simulink model "mainModel"  (R2024b)
settings: Solver=ode4  StartTime=0.0  StopTime=35000  FixedStep=0.1  RelTol=1e-3
values from neighbouring files (symbols this model uses):
  actuators = actuatorsConfig()    [main.m]
  constant = constantsConfig()    [main.m]
  control = controlConfig(data)    [main.m]
  MEKF = estimationConfig(sensors,simOpt)    [main.m]
  pert = pertConfig()    [main.m]
  sensors = sensorsConfig()    [main.m]
undefined symbols (not defined in the file or in its folder): Ab0, data, DiscIntNeverNeededParam, init
libraries: matrix_library x38, simulink x10, aerolibutil x7, simulink_extras x6, sharedtransform x1, dspinverses x1, dspfdesign x1, dspstat3 x1
(part 3 of 3)

== system mainModel/atmDrag/trash/Relative velocity body ==
  velRel_B : Inport
  om_B : Inport  Port=2
  rF_i : Inport  Port=3
  Add : Sum  Inputs=-+
  Cross Product : matrix_library/Cross Product
  Reshape : Reshape  OutputDimensionality=Row vector (2-D)
  Reshape1 : Reshape  OutputDimensionality=Row vector (2-D)
  vRelBody : Outport
  wires:
  velRel_B/1 -> Reshape/1
  Cross Product/1 -> Add/1
  om_B/1 -> Reshape1/1
  Reshape1/1 -> Cross Product/1
  rF_i/1 -> Cross Product/2
  Add/1 -> vRelBody/1
  Reshape/1 -> Add/2

== system mainModel/atmDrag/trash/Subsystem ==
  rho : Inport
  vRelBody : Inport  Port=2
  Nb_i : Inport  Port=3
  i : Inport  Port=4
  A_i : Inport  Port=5
  Assignment1 : Assignment  Commented=on  NumberOfDimensions=2  DiagnosticForDimensions=Warning  IndexOptions=Index vector (port),Assign all  Indices=1,1  OutputSizes=1,1
  Constant5 : Constant  Commented=on  Value=zeros(length(pert.drag.A), 1)  VectorParams1D=off
  Display2 : Display  Commented=on
  Dot Product : DotProduct  OutDataTypeStr=Inherit: Inherit via internal rule
  Gain : Gain  Gain=-1/2
  Gain1 : Gain  Gain=pert.drag.CD
  Gain2 : Gain  Gain=1e3
  Product : Product  Inputs=5
  Square : Math  Operator=square
  Subsystem Reference : Subsystem  ReferencedSubsystem=vecNorm
  F_i : Outport
  dotProd : Outport  Port=2
  wires:
  Product/1 -> F_i/1, Assignment1/2  "F_i"
  Subsystem Reference/1 -> Gain2/1
  rho/1 -> Gain/1
  Gain1/1 -> Product/1
  Dot Product/1 -> Product/4, dotProd/1
  Square/1 -> Product/2
  Gain/1 -> Gain1/1
  A_i/1 -> Product/5
  Nb_i/1 -> Dot Product/2
  vRelBody/1 -> Subsystem Reference/1
  Gain2/1 -> Square/1
  Constant5/1 -> Assignment1/1
  Assignment1/1 -> Display2/1
  i/1 -> Assignment1/3
  Subsystem Reference/2 -> Dot Product/1, Product/3

== system mainModel/attitudeDetermination_QUATERNION/QUEST V2/adjointMatrix ==
  A : Inport
  Reshape : Reshape  OutputDimensionality=Customize  OutputDimensions=[3,3]
  Subsystem Reference : Subsystem  ReferencedSubsystem=matrixCoFactors
  Out1 : Outport
  wires:
  Subsystem Reference/1 -> Reshape/1
  Reshape/1 -> Out1/1
  A/1 -> Subsystem Reference/1

== system mainModel/attitudeDetermination_QUATERNION/compute Kmatrix/Kmatrix ==
  S : Inport
  z : Inport  Port=2
  sigma : Inport  Port=3
  Constant : Constant  Value=eye(3)
  Minus : Sum  Inputs=+-
  Product : Product
  To Workspace4 : ToWorkspace  VariableName=K  SampleTime=-1
  Transpose : Math  Operator=transpose
  Vector Concatenate : Concatenate  Mode=Multidimensional array  ConcatenateDimension=2
  Vector Concatenate1 : Concatenate
  Vector Concatenate2 : Concatenate  Mode=Multidimensional array
  K : Outport
  wires:
  Constant/1 -> Product/2
  sigma/1 -> Vector Concatenate1/2, Product/1
  Product/1 -> Minus/2  "sigma*I"
  S/1 -> Minus/1  "Smatrix"
  Minus/1 -> Vector Concatenate/1  "S-sigma*I"
  z/1 -> Transpose/1, Vector Concatenate/2  "zVect"
  Transpose/1 -> Vector Concatenate1/1  "zVect^t"
  Vector Concatenate1/1 -> Vector Concatenate2/2  "[zVect^t  sigma]"
  Vector Concatenate/1 -> Vector Concatenate2/1  "[S-sigmaI  zVect]"
  Vector Concatenate2/1 -> To Workspace4/1, K/1  "Kmatrix"

== system mainModel/attitudeDetermination_QUATERNION/quest - shuster/compute optimal quaternion ==
  lambda : Inport
  sigma : Inport  Port=2
  k : Inport  Port=3
  Delta : Inport  Port=4
  S : Inport  Port=5
  z : Inport  Port=6
  Subsystem : Subsystem
  Subsystem Reference : Subsystem  ReferencedSubsystem=vecNorm
  Subsystem1 : Subsystem
  Subsystem2 : Subsystem
  Subsystem3 : Subsystem
  Terminator : Terminator
  Vector Concatenate : Concatenate
  q_est : Outport
  wires:
  Subsystem2/1(X) -> Vector Concatenate/1  "qv"
  Subsystem3/1(gamma) -> Vector Concatenate/2  "qw"
  lambda/1 -> Subsystem/1(lambda), Subsystem3/2(lambda), Subsystem1/1(lambda)
  sigma/1 -> Subsystem3/3(sigma), Subsystem/2(sigma), Subsystem1/2(sigma)
  k/1 -> Subsystem/3(k)
  S/1 -> Subsystem2/2(S)
  Subsystem/1(alpha) -> Subsystem3/1(alpha), Subsystem2/3(alpha)
  Subsystem1/1(beta) -> Subsystem2/4(beta)
  z/1 -> Subsystem2/1(z)
  Delta/1 -> Subsystem3/4(Delta)
  Vector Concatenate/1 -> Subsystem Reference/1
  Subsystem Reference/2 -> q_est/1
  Subsystem Reference/1 -> Terminator/1

== system mainModel/attitudeDetermination_QUATERNION/quest - shuster/mewton method step-two ==
  lambda1 : Inport
  sigma : Inport  Port=2
  a : Inport  Port=3
  b : Inport  Port=4
  c : Inport  Port=5
  d : Inport  Port=6
  Abs : Abs  Commented=on  SaturateOnIntegerOverflow=off
  Compare To Constant : simulink/Logic and Bit Operations/Compare To Constant  Commented=on  relop=>=  const=5  OutDataTypeStr=boolean
  Scope : Scope  Commented=on
  Scope1 : Scope  Commented=on
  Switch : Switch  Commented=on  Criteria=u2 > Threshold  SaturateOnIntegerOverflow=off  InputSameDT=off
  characteristic polynomial derivative1 : Subsystem
  characteristic polynomial1 : Subsystem
  "newton method " : Subsystem
  lambda : Outport
  wires:
  lambda1/1 -> characteristic polynomial derivative1/1(lambda), characteristic polynomial1/1(lambda1), Switch/3, "newton method "/1(lambda1)
  b/1 -> characteristic polynomial derivative1/3(b), characteristic polynomial1/4(b)
  "newton method "/1(lambda) -> lambda/1, Switch/1  "lambda"
  characteristic polynomial derivative1/1(p'(lambda)) -> Abs/1, "newton method "/3(p'(lambda))
  characteristic polynomial1/1(p(lambda)) -> "newton method "/2(p(lambda))
  c/1 -> characteristic polynomial derivative1/4(c), characteristic polynomial1/5(c)
  d/1 -> characteristic polynomial1/6(d)
  sigma/1 -> characteristic polynomial1/2(sigma)
  a/1 -> characteristic polynomial derivative1/2(a), characteristic polynomial1/3(a)
  Compare To Constant/1 -> Scope1/1, Switch/2
  Switch/1 -> ?
  Abs/1 -> Scope/1, Compare To Constant/1

== system mainModel/attitudeDetermination_QUATERNION/quest - shuster/newton method step-one ==
  lambda : Inport
  sigma : Inport  Port=2
  a : Inport  Port=3
  b : Inport  Port=4
  c : Inport  Port=5
  d : Inport  Port=6
  characteristic polynomial : Subsystem
  characteristic polynomial derivative : Subsystem
  newton method step-one : Subsystem
  lambda1 : Outport
  wires:
  a/1 -> characteristic polynomial derivative/2(a), characteristic polynomial/3(a)
  newton method step-one/1(lambda1) -> lambda1/1  "lambda1"
  c/1 -> characteristic polynomial/5(c), characteristic polynomial derivative/4(c)
  sigma/1 -> characteristic polynomial/2(sigma)
  characteristic polynomial derivative/1(p'(lambda)) -> newton method step-one/2(p'(lambda))
  d/1 -> characteristic polynomial/6(d)
  characteristic polynomial/1(p(lambda)) -> newton method step-one/1(p(lambda))
  lambda/1 -> characteristic polynomial/1(lambda), characteristic polynomial derivative/1(lambda)
  b/1 -> characteristic polynomial derivative/3(b), characteristic polynomial/4(b)

== system mainModel/attitudeDetermination_QUATERNION/quest - shuster/shuster parameters ==
  S : Inport
  z : Inport  Port=2
  Sigma : Subsystem
  compute Delta : Subsystem
  compute a : Subsystem
  compute b : Subsystem
  compute c : Subsystem
  compute d : Subsystem
  compute k : Subsystem
  a : Outport
  b : Outport  Port=2
  c : Outport  Port=3
  d : Outport  Port=4
  sigma : Outport  Port=5
  k : Outport  Port=6
  Delta : Outport  Port=7
  wires:
  compute k/1(k) -> compute a/2(k), k/1
  S/1 -> compute d/1(S), compute c/3(S), compute Delta/1(S), compute k/1(S), Sigma/1(S)
  compute c/1(c) -> c/1  "c"
  z/1 -> compute d/2(z), compute c/2(z), compute b/2(z)
  compute Delta/1(Delta) -> Delta/1, compute c/1(Delta)
  compute a/1(a) -> a/1  "a"
  Sigma/1(sigma) -> compute b/1(sigma), sigma/1, compute a/1(sigma)  "sigma"
  compute b/1(b) -> b/1  "b"
  compute d/1(d) -> d/1  "d"

== system mainModel/starSensorModel/star mapping/keep3 ==
  In1 : Inport
  Abs : Abs  SaturateOnIntegerOverflow=off
  Memory : Memory  InheritSampleTime=on
  Sum of Elements1 : Sum  Inputs=+
  Switch : Switch  Criteria=u2 > Threshold  SaturateOnIntegerOverflow=off  InputSameDT=off
  s_N4 : Outport
  wires:
  Switch/1 -> s_N4/1, Memory/1
  Abs/1 -> Switch/2
  Memory/1 -> Switch/1, Sum of Elements1/1
  Sum of Elements1/1 -> Abs/1
  In1/1 -> Switch/3

== system mainModel/MEKF ESTIMATION/MEASUREMENT/KALMAN GAIN/avoid sing ==
  S : Inport
  Add : Sum
  Constant : Constant  Value=eye(6)*1e-12
  S_ : Outport
  wires:
  S/1 -> Add/2
  Constant/1 -> Add/1
  Add/1 -> S_/1

== system mainModel/MEKF ESTIMATION/MEASUREMENT/SENSITIVITY MATRIX/skewMatrix ==
  note: b_pred_skew = [0 , -b_pred(3) , b_pred(2) ;
      | b_pred(3) , 0 , -b_pred(1) ;
      | -b_pred(2) , b_pred(1) , 0 ];
  vect : Inport
  Constant : Constant  Value=0
  Demux : Demux  Outputs=3
  Gain : Gain  Gain=-1
  Gain1 : Gain  Gain=-1
  Gain2 : Gain  Gain=-1
  Reshape : Reshape  OutputDimensionality=Row vector (2-D)
  Reshape1 : Reshape  OutputDimensionality=Row vector (2-D)
  Reshape2 : Reshape  OutputDimensionality=Row vector (2-D)
  Vector Concatenate : Concatenate  NumInputs=3
  Vector Concatenate1 : Concatenate  NumInputs=3
  Vector Concatenate2 : Concatenate  NumInputs=3
  Vector Concatenate3 : Concatenate  NumInputs=3  Mode=Multidimensional array
  skew : Outport
  wires:
  Demux/1 -> Vector Concatenate2/2, Gain1/1  "x"
  Gain2/1 -> Vector Concatenate2/1
  Vector Concatenate1/1 -> Reshape1/1
  Constant/1 -> Vector Concatenate/1, Vector Concatenate1/2, Vector Concatenate2/3
  Vector Concatenate3/1 -> skew/1
  Gain/1 -> Vector Concatenate/2
  Demux/2 -> Gain2/1, Vector Concatenate/3  "y"
  Gain1/1 -> Vector Concatenate1/3
  Vector Concatenate2/1 -> Reshape2/1
  Reshape2/1 -> Vector Concatenate3/3
  Demux/3 -> Gain/1, Vector Concatenate1/1  "z"
  vect/1 -> Demux/1
  Reshape/1 -> Vector Concatenate3/1
  Vector Concatenate/1 -> Reshape/1
  Reshape1/1 -> Vector Concatenate3/2

== system mainModel/MEKF ESTIMATION/PREDICTION/STATE PROPAGATION/QUATERNION KINEMATICS ==
  q_corr : Inport
  w_corr : Inport  Port=2
  Add2 : Sum
  Constant : Constant  Value=0
  Gain : Gain  Gain=1/2
  Gain1 : Gain  Commented=on  Gain=0.5
  Gain2 : Gain  Gain=MEKF.dt
  Reshape : Reshape  OutputDimensionality=Row vector (2-D)
  Subsystem Reference : Subsystem  ReferencedSubsystem=vecNorm
  Terminator : Terminator
  Vector Concatenate : Concatenate
  q_corr x w_corr_quat : aerolibutil/Quaternion Multiplication
  quatMolt : Subsystem  Commented=on
  q_pred : Outport
  wires:
  Constant/1 -> Vector Concatenate/1
  w_corr/1 -> Vector Concatenate/2
  Vector Concatenate/1 -> quatMolt/2(In2), q_corr x w_corr_quat/2  "w_corr_quat"
  Gain2/1 -> Add2/2
  Add2/1 -> Subsystem Reference/1  "q_pred"
  q_corr/1 -> Reshape/1  "q_corr"
  Gain/1 -> Gain2/1  "qDot_pred"
  q_corr x w_corr_quat/1 -> Gain/1
  Subsystem Reference/2 -> q_pred/1
  Subsystem Reference/1 -> Terminator/1
  Reshape/1 -> Add2/1, quatMolt/1(In1), q_corr x w_corr_quat/1
  quatMolt/1(quaternions) -> Gain1/1

== system mainModel/MEKF ESTIMATION/PREDICTION/STATE PROPAGATION/SYSTEM DYNAMICS ==
  w_corr : Inport
  J : Inport  Port=2
  hWheel : Inport  Port=3
  hDotWheel : Inport  Port=4
  distTq : Inport  Port=5
  controlTq : Inport  Port=6
  Add : Sum
  Add1 : Sum  Inputs=++++
  Add2 : Sum
  Cross Product : matrix_library/Cross Product
  Cross Product1 : matrix_library/Cross Product
  Gain : Gain  Gain=-1
  Gain1 : Gain  Gain=-1
  Gain2 : Gain  Gain=MEKF.dt
  Gain3 : Gain  Gain=inv(data.Imatrix)  Multiplication=Matrix(K*u)
  Product : Product  Multiplication=Matrix(*)
  Reshape : Reshape  OutputDimensionality=Column vector (2-D)
  Reshape4 : Reshape
  w_pred : Outport
  wires:
  Product/1 -> Cross Product/2  "J*w"
  Add1/1 -> Gain3/1  "totalTq"
  Gain2/1 -> Add2/2
  J/1 -> Product/1  "J"
  w_corr/1 -> Reshape/1  "w_corr"
  Gain3/1 -> Gain2/1  "wDot_pred"
  Cross Product1/1 -> Add/2  "w x h"
  Add/1 -> Gain/1  "gyro"
  Gain/1 -> Reshape4/1
  Cross Product/1 -> Add/1  "w x Jw"
  Add2/1 -> w_pred/1  "w_pred"
  hDotWheel/1 -> Gain1/1  "hDot"
  hWheel/1 -> Cross Product1/2  "h"
  Reshape/1 -> Add2/1, Cross Product/1, Product/2, Cross Product1/1
  controlTq/1 -> Add1/4
  distTq/1 -> Add1/3
  Gain1/1 -> Add1/2
  Reshape4/1 -> Add1/1

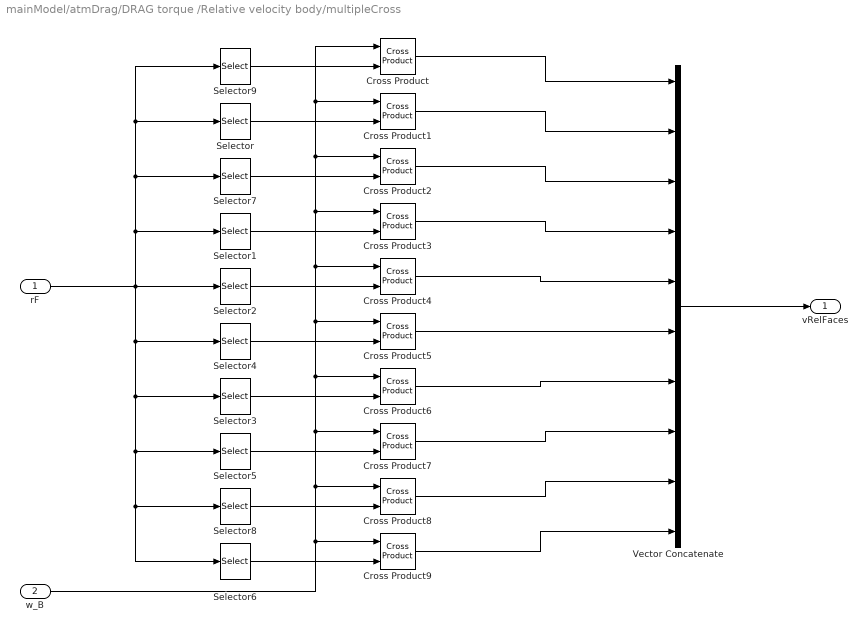
== system mainModel/atmDrag/DRAG torque /Relative velocity body/multipleCross ==
  rF : Inport
  w_B : Inport  Port=2
  Cross Product{,1..9} (10 alike) : matrix_library/Cross Product
  Selector : Selector  NumberOfDimensions=2  InputPortWidth=3  IndexOptions=Index vector (dialog),Select all  Indices=2,[1:3]  OutputSizes=1,1
  Selector1 : Selector  NumberOfDimensions=2  InputPortWidth=3  IndexOptions=Index vector (dialog),Select all  Indices=4,[1:3]  OutputSizes=1,1
  Selector2 : Selector  NumberOfDimensions=2  InputPortWidth=3  IndexOptions=Index vector (dialog),Select all  Indices=5,[1:3]  OutputSizes=1,1
  Selector3 : Selector  NumberOfDimensions=2  InputPortWidth=3  IndexOptions=Index vector (dialog),Select all  Indices=7,[1:3]  OutputSizes=1,1
  Selector4 : Selector  NumberOfDimensions=2  InputPortWidth=3  IndexOptions=Index vector (dialog),Select all  Indices=6,[1:3]  OutputSizes=1,1
  Selector5 : Selector  NumberOfDimensions=2  InputPortWidth=3  IndexOptions=Index vector (dialog),Select all  Indices=8,[1:3]  OutputSizes=1,1
  Selector6 : Selector  NumberOfDimensions=2  InputPortWidth=3  IndexOptions=Index vector (dialog),Select all  Indices=10,[1:3]  OutputSizes=1,1
  Selector7 : Selector  NumberOfDimensions=2  InputPortWidth=3  IndexOptions=Index vector (dialog),Select all  Indices=3,[1:3]  OutputSizes=1,1
  Selector8 : Selector  NumberOfDimensions=2  InputPortWidth=3  IndexOptions=Index vector (dialog),Select all  Indices=9,[1:3]  OutputSizes=1,1
  Selector9 : Selector  NumberOfDimensions=2  InputPortWidth=3  IndexOptions=Index vector (dialog),Select all  Indices=1,[1:3]  OutputSizes=1,1
  Vector Concatenate : Concatenate  NumInputs=10  Mode=Multidimensional array
  vRelFaces : Outport
  wires:
  rF/1 -> Selector9/1, Selector/1, Selector7/1, Selector1/1, Selector2/1, Selector6/1, Selector8/1, Selector5/1, Selector3/1, Selector4/1
  Vector Concatenate/1 -> vRelFaces/1
  w_B/1 -> Cross Product6/1, Cross Product/1, Cross Product1/1, Cross Product2/1, Cross Product3/1, Cross Product4/1, Cross Product5/1, Cross Product7/1, Cross Product8/1, Cross Product9/1
  Selector9/1 -> Cross Product/2
  Selector/1 -> Cross Product1/2
  Selector7/1 -> Cross Product2/2
  Selector1/1 -> Cross Product3/2
  Selector2/1 -> Cross Product4/2
  Selector4/1 -> Cross Product5/2
  Selector3/1 -> Cross Product6/2
  Selector5/1 -> Cross Product7/2
  Selector8/1 -> Cross Product8/2
  Selector6/1 -> Cross Product9/2
  Cross Product9/1 -> Vector Concatenate/10
  Cross Product8/1 -> Vector Concatenate/9
  Cross Product7/1 -> Vector Concatenate/8
  Cross Product6/1 -> Vector Concatenate/7
  Cross Product5/1 -> Vector Concatenate/6
  Cross Product4/1 -> Vector Concatenate/5
  Cross Product3/1 -> Vector Concatenate/4
  Cross Product2/1 -> Vector Concatenate/3
  Cross Product/1 -> Vector Concatenate/1
  Cross Product1/1 -> Vector Concatenate/2

== system mainModel/atmDrag/DRAG torque /Relative velocity body/vecSum ==
  vRel_B : Inport
  vRelFaces : Inport  Port=2
  Minus : Sum
  Minus1 : Sum
  Minus2 : Sum
  Selector : Selector  InputPortWidth=3  IndexOptions=Index vector (dialog)  Indices=1  OutputSizes=1
  Selector1 : Selector  InputPortWidth=3  IndexOptions=Index vector (dialog)  Indices=2  OutputSizes=1
  Selector2 : Selector  InputPortWidth=3  IndexOptions=Index vector (dialog)  Indices=3  OutputSizes=1
  Selector3 : Selector  NumberOfDimensions=2  InputPortWidth=3  IndexOptions=Select all,Index vector (dialog)  Indices=[1 3],1  OutputSizes=1,1
  Selector4 : Selector  NumberOfDimensions=2  InputPortWidth=3  IndexOptions=Select all,Index vector (dialog)  Indices=[1 3],2  OutputSizes=1,1
  Selector5 : Selector  NumberOfDimensions=2  InputPortWidth=3  IndexOptions=Select all,Index vector (dialog)  Indices=[1 3],3  OutputSizes=1,1
  Vector Concatenate : Concatenate  NumInputs=3  Mode=Multidimensional array  ConcatenateDimension=2
  prod : Outport
  wires:
  Minus/1 -> Vector Concatenate/3
  Minus2/1 -> Vector Concatenate/1
  Selector3/1 -> Minus2/2
  Selector4/1 -> Minus1/2
  vRelFaces/1 -> Selector5/1, Selector3/1, Selector4/1
  Minus1/1 -> Vector Concatenate/2
  Selector5/1 -> Minus/2
  Vector Concatenate/1 -> prod/1
  Selector2/1 -> Minus/1
  vRel_B/1 -> Selector/1, Selector1/1, Selector2/1
  Selector1/1 -> Minus1/1
  Selector/1 -> Minus2/1

== system mainModel/atmDrag/DRAG torque /dragForce/multipleDotProd ==
  Nbvect : Inport
  vers : Inport  Port=2
  Constant : Constant  Value=0
  Product : Product
  Sum of Elements : Sum  Inputs=+  CollapseMode=Specified dimension  CollapseDim=2
  Switch : Switch  SaturateOnIntegerOverflow=off  InputSameDT=off
  dotSmooth : Subsystem
  visionVec : Outport
  wires:
  Nbvect/1 -> Product/1
  vers/1 -> Product/2
  Product/1 -> Sum of Elements/1
  Constant/1 -> Switch/3
  Sum of Elements/1 -> dotSmooth/1(dot), Switch/2, Switch/1
  dotSmooth/1(dotSmooth) -> visionVec/1

== system mainModel/atmDrag/DRAG torque /dragForce/multipleVecNorm ==
  vRelBody : Inport
  Sqrt : Sqrt
  Square : Math  Operator=square
  Sum of Elements : Sum  Inputs=+  CollapseMode=Specified dimension  CollapseDim=2
  normVec : Outport
  wires:
  Square/1 -> Sum of Elements/1
  vRelBody/1 -> Square/1
  Sum of Elements/1 -> Sqrt/1
  Sqrt/1 -> normVec/1

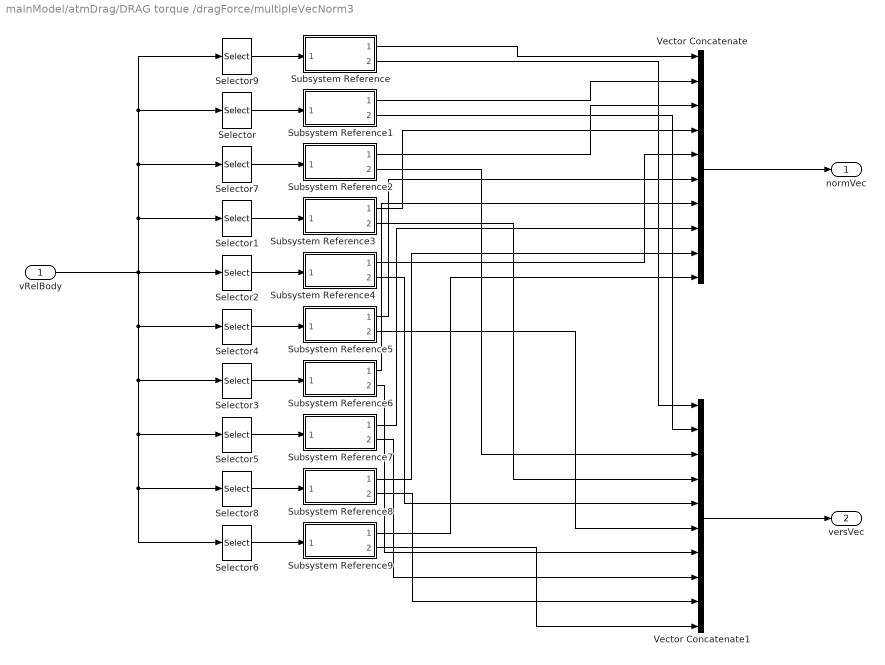
== system mainModel/atmDrag/DRAG torque /dragForce/multipleVecNorm3 ==
  vRelBody : Inport
  Selector : Selector  NumberOfDimensions=2  InputPortWidth=3  IndexOptions=Index vector (dialog),Select all  Indices=2,[1:3]  OutputSizes=1,1
  Selector1 : Selector  NumberOfDimensions=2  InputPortWidth=3  IndexOptions=Index vector (dialog),Select all  Indices=4,[1:3]  OutputSizes=1,1
  Selector2 : Selector  NumberOfDimensions=2  InputPortWidth=3  IndexOptions=Index vector (dialog),Select all  Indices=5,[1:3]  OutputSizes=1,1
  Selector3 : Selector  NumberOfDimensions=2  InputPortWidth=3  IndexOptions=Index vector (dialog),Select all  Indices=7,[1:3]  OutputSizes=1,1
  Selector4 : Selector  NumberOfDimensions=2  InputPortWidth=3  IndexOptions=Index vector (dialog),Select all  Indices=6,[1:3]  OutputSizes=1,1
  Selector5 : Selector  NumberOfDimensions=2  InputPortWidth=3  IndexOptions=Index vector (dialog),Select all  Indices=8,[1:3]  OutputSizes=1,1
  Selector6 : Selector  NumberOfDimensions=2  InputPortWidth=3  IndexOptions=Index vector (dialog),Select all  Indices=10,[1:3]  OutputSizes=1,1
  Selector7 : Selector  NumberOfDimensions=2  InputPortWidth=3  IndexOptions=Index vector (dialog),Select all  Indices=3,[1:3]  OutputSizes=1,1
  Selector8 : Selector  NumberOfDimensions=2  InputPortWidth=3  IndexOptions=Index vector (dialog),Select all  Indices=9,[1:3]  OutputSizes=1,1
  Selector9 : Selector  NumberOfDimensions=2  InputPortWidth=3  IndexOptions=Index vector (dialog),Select all  Indices=1,[1:3]  OutputSizes=1,1
  Subsystem Reference{,1..9} (10 alike) : Subsystem  ReferencedSubsystem=vecNorm
  Vector Concatenate : Concatenate  NumInputs=10  Mode=Multidimensional array
  Vector Concatenate1 : Concatenate  NumInputs=10  Mode=Multidimensional array
  normVec : Outport
  versVec : Outport  Port=2
  wires:
  Vector Concatenate/1 -> normVec/1
  vRelBody/1 -> Selector9/1, Selector/1, Selector7/1, Selector1/1, Selector2/1, Selector6/1, Selector8/1, Selector5/1, Selector3/1, Selector4/1
  Selector9/1 -> Subsystem Reference/1
  Selector/1 -> Subsystem Reference1/1
  Selector1/1 -> Subsystem Reference3/1
  Selector7/1 -> Subsystem Reference2/1
  Selector4/1 -> Subsystem Reference5/1
  Selector3/1 -> Subsystem Reference6/1
  Selector5/1 -> Subsystem Reference7/1
  Selector2/1 -> Subsystem Reference4/1
  Selector6/1 -> Subsystem Reference9/1
  Selector8/1 -> Subsystem Reference8/1
  Vector Concatenate1/1 -> versVec/1
  Subsystem Reference/1 -> Vector Concatenate/1
  Subsystem Reference1/1 -> Vector Concatenate/2
  Subsystem Reference2/1 -> Vector Concatenate/3
  Subsystem Reference3/1 -> Vector Concatenate/4
  Subsystem Reference4/1 -> Vector Concatenate/5
  Subsystem Reference5/1 -> Vector Concatenate/6
  Subsystem Reference6/1 -> Vector Concatenate/7
  Subsystem Reference7/1 -> Vector Concatenate/8
  Subsystem Reference8/1 -> Vector Concatenate/9
  Subsystem Reference9/1 -> Vector Concatenate/10
  Subsystem Reference9/2 -> Vector Concatenate1/10
  Subsystem Reference8/2 -> Vector Concatenate1/9
  Subsystem Reference7/2 -> Vector Concatenate1/8
  Subsystem Reference6/2 -> Vector Concatenate1/7
  Subsystem Reference5/2 -> Vector Concatenate1/6
  Subsystem Reference4/2 -> Vector Concatenate1/5
  Subsystem Reference3/2 -> Vector Concatenate1/4
  Subsystem Reference2/2 -> Vector Concatenate1/3
  Subsystem Reference1/2 -> Vector Concatenate1/2
  Subsystem Reference/2 -> Vector Concatenate1/1

== system mainModel/atmDrag/DRAG torque /dragForce/multipleVersVec ==
  vRelBody : Inport
  normVec : Inport  Port=2
  Divide : Product  Inputs=*/
  Divide1 : Product  Inputs=*/
  Divide2 : Product  Inputs=*/
  Selector : Selector  NumberOfDimensions=2  InputPortWidth=3  IndexOptions=Select all,Index vector (dialog)  Indices=[1 3],1  OutputSizes=1,1
  Selector1 : Selector  NumberOfDimensions=2  InputPortWidth=3  IndexOptions=Select all,Index vector (dialog)  Indices=[1 3],2  OutputSizes=1,1
  Selector2 : Selector  NumberOfDimensions=2  InputPortWidth=3  IndexOptions=Select all,Index vector (dialog)  Indices=[1 3],3  OutputSizes=1,1
  Vector Concatenate : Concatenate  NumInputs=3  Mode=Multidimensional array  ConcatenateDimension=2
  versVec : Outport
  wires:
  normVec/1 -> Divide/2, Divide2/2, Divide1/2
  vRelBody/1 -> Selector2/1, Selector/1, Selector1/1
  Selector2/1 -> Divide/1
  Selector1/1 -> Divide1/1
  Selector/1 -> Divide2/1
  Divide1/1 -> Vector Concatenate/2
  Divide2/1 -> Vector Concatenate/1
  Divide/1 -> Vector Concatenate/3
  Vector Concatenate/1 -> versVec/1

== system mainModel/atmDrag/DRAG torque /dragForce/vecProd ==
  constVec : Inport
  versVec : Inport  Port=2
  Divide : Product  Inputs=**
  Divide1 : Product  Inputs=**
  Divide2 : Product  Inputs=**
  Selector : Selector  NumberOfDimensions=2  InputPortWidth=3  IndexOptions=Select all,Index vector (dialog)  Indices=[1 3],1  OutputSizes=1,1
  Selector1 : Selector  NumberOfDimensions=2  InputPortWidth=3  IndexOptions=Select all,Index vector (dialog)  Indices=[1 3],2  OutputSizes=1,1
  Selector2 : Selector  NumberOfDimensions=2  InputPortWidth=3  IndexOptions=Select all,Index vector (dialog)  Indices=[1 3],3  OutputSizes=1,1
  Vector Concatenate : Concatenate  NumInputs=3  Mode=Multidimensional array  ConcatenateDimension=2
  Fvect : Outport
  wires:
  Divide2/1 -> Vector Concatenate/1
  Vector Concatenate/1 -> Fvect/1
  Divide/1 -> Vector Concatenate/3
  constVec/1 -> Divide/2, Divide2/2, Divide1/2
  Selector/1 -> Divide2/1
  Selector2/1 -> Divide/1
  versVec/1 -> Selector2/1, Selector1/1, Selector/1
  Selector1/1 -> Divide1/1
  Divide1/1 -> Vector Concatenate/2

== system mainModel/atmDrag/DRAG torque /vecCrossOld/Subsystem ==
  Fvect : Inport
  Selector : Selector  NumberOfDimensions=2  InputPortWidth=3  IndexOptions=Index vector (dialog),Select all  Indices=1,1  OutputSizes=1,1
  Selector1 : Selector  NumberOfDimensions=2  InputPortWidth=3  IndexOptions=Index vector (dialog),Select all  Indices=2,1  OutputSizes=1,1
  Selector2 : Selector  NumberOfDimensions=2  InputPortWidth=3  IndexOptions=Index vector (dialog),Select all  Indices=3,1  OutputSizes=1,1
  Selector3 : Selector  NumberOfDimensions=2  InputPortWidth=3  IndexOptions=Index vector (dialog),Select all  Indices=4,1  OutputSizes=1,1
  Selector4 : Selector  NumberOfDimensions=2  InputPortWidth=3  IndexOptions=Index vector (dialog),Select all  Indices=5,1  OutputSizes=1,1
  Selector5 : Selector  NumberOfDimensions=2  InputPortWidth=3  IndexOptions=Index vector (dialog),Select all  Indices=6,1  OutputSizes=1,1
  Selector6 : Selector  NumberOfDimensions=2  InputPortWidth=3  IndexOptions=Index vector (dialog),Select all  Indices=7,1  OutputSizes=1,1
  Selector7 : Selector  NumberOfDimensions=2  InputPortWidth=3  IndexOptions=Index vector (dialog),Select all  Indices=8,1  OutputSizes=1,1
  Selector8 : Selector  NumberOfDimensions=2  InputPortWidth=3  IndexOptions=Index vector (dialog),Select all  Indices=9,1  OutputSizes=1,1
  Selector9 : Selector  NumberOfDimensions=2  InputPortWidth=3  IndexOptions=Index vector (dialog),Select all  Indices=10,1  OutputSizes=1,1
  F1 : Outport
  F2 : Outport  Port=2
  F3 : Outport  Port=3
  F4 : Outport  Port=4
  F5 : Outport  Port=5
  F6 : Outport  Port=6
  F7 : Outport  Port=7
  F8 : Outport  Port=8
  F9 : Outport  Port=9
  F10 : Outport  Port=10
  wires:
  Selector5/1 -> F6/1  "F6"
  Fvect/1 -> Selector5/1, Selector9/1, Selector8/1, Selector7/1, Selector6/1, Selector1/1, Selector/1, Selector2/1, Selector3/1, Selector4/1
  Selector/1 -> F1/1  "F1"
  Selector4/1 -> F5/1  "F5"
  Selector8/1 -> F9/1  "F9"
  Selector3/1 -> F4/1  "F4"
  Selector1/1 -> F2/1  "F2"
  Selector7/1 -> F8/1  "F8"
  Selector2/1 -> F3/1  "F3"
  Selector9/1 -> F10/1  "F10"
  Selector6/1 -> F7/1  "F7"

== system mainModel/atmDrag/DRAG torque /vecCrossOld/Subsystem1 ==
  In1 : Inport
  Selector : Selector  NumberOfDimensions=2  InputPortWidth=3  IndexOptions=Index vector (dialog),Select all  Indices=1,1  OutputSizes=1,1
  Selector1 : Selector  NumberOfDimensions=2  InputPortWidth=3  IndexOptions=Index vector (dialog),Select all  Indices=2,1  OutputSizes=1,1
  Selector2 : Selector  NumberOfDimensions=2  InputPortWidth=3  IndexOptions=Index vector (dialog),Select all  Indices=3,1  OutputSizes=1,1
  Selector3 : Selector  NumberOfDimensions=2  InputPortWidth=3  IndexOptions=Index vector (dialog),Select all  Indices=4,1  OutputSizes=1,1
  Selector4 : Selector  NumberOfDimensions=2  InputPortWidth=3  IndexOptions=Index vector (dialog),Select all  Indices=5,1  OutputSizes=1,1
  Selector5 : Selector  NumberOfDimensions=2  InputPortWidth=3  IndexOptions=Index vector (dialog),Select all  Indices=6,1  OutputSizes=1,1
  Selector6 : Selector  NumberOfDimensions=2  InputPortWidth=3  IndexOptions=Index vector (dialog),Select all  Indices=7,1  OutputSizes=1,1
  Selector7 : Selector  NumberOfDimensions=2  InputPortWidth=3  IndexOptions=Index vector (dialog),Select all  Indices=8,1  OutputSizes=1,1
  Selector8 : Selector  NumberOfDimensions=2  InputPortWidth=3  IndexOptions=Index vector (dialog),Select all  Indices=9,1  OutputSizes=1,1
  Selector9 : Selector  NumberOfDimensions=2  InputPortWidth=3  IndexOptions=Index vector (dialog),Select all  Indices=10,1  OutputSizes=1,1
  rF1 : Outport
  rF2 : Outport  Port=2
  rF3 : Outport  Port=3
  rF4 : Outport  Port=4
  rF5 : Outport  Port=5
  rF6 : Outport  Port=6
  rF7 : Outport  Port=7
  rF8 : Outport  Port=8
  rF9 : Outport  Port=9
  rF10 : Outport  Port=10
  wires:
  Selector9/1 -> rF10/1  "rF10"
  Selector8/1 -> rF9/1  "rF9"
  Selector7/1 -> rF8/1  "rF8"
  Selector6/1 -> rF7/1  "rF7"
  Selector2/1 -> rF3/1  "rF3"
  Selector5/1 -> rF6/1  "rF6"
  Selector4/1 -> rF5/1  "rF5"
  Selector/1 -> rF1/1  "rF1"
  Selector1/1 -> rF2/1  "rF2"
  In1/1 -> Selector5/1, Selector9/1, Selector8/1, Selector7/1, Selector6/1, Selector1/1, Selector/1, Selector2/1, Selector3/1, Selector4/1  "rFvect"
  Selector3/1 -> rF4/1  "rF4"

== system mainModel/attitudeDetermination_QUATERNION/quest - shuster/compute optimal quaternion/Subsystem ==
  lambda : Inport
  sigma : Inport  Port=2
  k : Inport  Port=3
  Add : Sum  Inputs=+-+
  Square : Math  Operator=square
  Square1 : Math  Operator=square
  alpha : Outport
  wires:
  sigma/1 -> Square1/1
  lambda/1 -> Square/1
  Square1/1 -> Add/2
  Square/1 -> Add/1
  k/1 -> Add/3
  Add/1 -> alpha/1

== system mainModel/attitudeDetermination_QUATERNION/quest - shuster/compute optimal quaternion/Subsystem1 ==
  lambda : Inport
  sigma : Inport  Port=2
  Minus : Sum  Inputs=+-
  beta : Outport
  wires:
  lambda/1 -> Minus/1
  sigma/1 -> Minus/2
  Minus/1 -> beta/1

== system mainModel/attitudeDetermination_QUATERNION/quest - shuster/compute optimal quaternion/Subsystem2 ==
  z : Inport
  S : Inport  Port=2
  alpha : Inport  Port=3
  beta : Inport  Port=4
  (-) * z : Product  Multiplication=Matrix(*)
  Add : Sum  Inputs=+++
  Constant : Constant  Value=eye(3)
  Product : Product
  Product1 : Product
  S * S : Product  Multiplication=Matrix(*)
  X : Outport
  wires:
  alpha/1 -> Product/1
  Constant/1 -> Product/2
  beta/1 -> Product1/2
  S/1 -> S * S/1, S * S/2, Product1/1
  Product1/1 -> Add/2
  S * S/1 -> Add/1
  Product/1 -> Add/3
  Add/1 -> (-) * z/1
  z/1 -> (-) * z/2
  (-) * z/1 -> X/1

== system mainModel/attitudeDetermination_QUATERNION/quest - shuster/compute optimal quaternion/Subsystem3 ==
  alpha : Inport
  lambda : Inport  Port=2
  sigma : Inport  Port=3
  Delta : Inport  Port=4
  Add : Sum
  Minus : Sum  Inputs=+-
  Product : Product
  gamma : Outport
  wires:
  sigma/1 -> Add/1
  lambda/1 -> Add/2
  alpha/1 -> Product/1
  Add/1 -> Product/2
  Product/1 -> Minus/1
  Delta/1 -> Minus/2
  Minus/1 -> gamma/1

== system mainModel/attitudeDetermination_QUATERNION/quest - shuster/mewton method step-two/characteristic polynomial derivative1 ==
  lambda : Inport
  a : Inport  Port=2
  b : Inport  Port=3
  c : Inport  Port=4
  Add : Sum  Inputs=+++
  Add1 : Sum
  Constant1 : Constant  Value=3
  Gain : Gain  Gain=-2
  Gain1 : Gain  Gain=-1
  Gain2 : Gain  Gain=4
  Power : Math  Operator=pow
  Product : Product
  p'(lambda) : Outport
  wires:
  Constant1/1 -> Power/2
  a/1 -> Add1/1  "a"
  b/1 -> Add1/2  "b"
  Product/1 -> Gain/1
  Gain/1 -> Add/2
  Power/1 -> Gain2/1
  Add1/1 -> Product/2
  c/1 -> Gain1/1  "c"
  lambda/1 -> Power/1, Product/1  "lambda"
  Gain1/1 -> Add/3
  Add/1 -> p'(lambda)/1
  Gain2/1 -> Add/1

== system mainModel/attitudeDetermination_QUATERNION/quest - shuster/mewton method step-two/characteristic polynomial1 ==
  lambda1 : Inport
  sigma : Inport  Port=2
  a : Inport  Port=3
  b : Inport  Port=4
  c : Inport  Port=5
  d : Inport  Port=6
  Add : Sum  Inputs=++++
  Add1 : Sum
  Add2 : Sum  Inputs=+++
  Constant1 : Constant  Value=4
  Constant2 : Constant  Value=2
  Gain : Gain  Gain=-1
  Gain1 : Gain  Gain=-1
  Gain2 : Gain  Gain=-1
  Power : Math  Operator=pow
  Power1 : Math  Operator=pow
  Product{,1..3} (4 alike) : Product
  p(lambda) : Outport
  wires:
  Constant1/1 -> Power/2
  Constant2/1 -> Power1/2
  a/1 -> Product3/1, Add1/1  "a"
  b/1 -> Add1/2, Product3/2  "b"
  Power1/1 -> Product/1
  Product/1 -> Gain/1
  Gain/1 -> Add/2
  Power/1 -> Add/1
  Add1/1 -> Product/2
  c/1 -> Product1/2, Product2/1  "c"
  Product1/1 -> Gain1/1
  lambda1/1 -> Product1/1, Power1/1, Power/1  "lambda"
  Gain1/1 -> Add/3
  Add2/1 -> Add/4
  d/1 -> Gain2/1
  Gain2/1 -> Add2/3
  sigma/1 -> Product2/2
  Product2/1 -> Add2/2
  Product3/1 -> Add2/1
  Add/1 -> p(lambda)/1

== system mainModel/attitudeDetermination_QUATERNION/quest - shuster/mewton method step-two/newton method  ==
  note: lambda0 can be setted as SIGMA only if two step newton is implemented
  lambda1 : Inport
  p(lambda) : Inport  Port=2
  p'(lambda) : Inport  Port=3
  Divide : Product  Inputs=*/
  Sum : Sum  Inputs=+-
  lambda : Outport
  wires:
  Sum/1 -> lambda/1
  p(lambda)/1 -> Divide/1
  p'(lambda)/1 -> Divide/2
  Divide/1 -> Sum/2
  lambda1/1 -> Sum/1

== system mainModel/attitudeDetermination_QUATERNION/quest - shuster/newton method step-one/characteristic polynomial ==
  lambda : Inport
  sigma : Inport  Port=2
  a : Inport  Port=3
  b : Inport  Port=4
  c : Inport  Port=5
  d : Inport  Port=6
  Add : Sum  Inputs=++++
  Add1 : Sum
  Add2 : Sum  Inputs=+++
  Constant1 : Constant  Value=4
  Constant2 : Constant  Value=2
  Gain : Gain  Gain=-1
  Gain1 : Gain  Gain=-1
  Gain2 : Gain  Gain=-1
  Power : Math  Operator=pow
  Power1 : Math  Operator=pow
  Product{,1..3} (4 alike) : Product
  p(lambda) : Outport
  wires:
  Constant1/1 -> Power/2
  Constant2/1 -> Power1/2
  a/1 -> Product3/1, Add1/1  "a"
  b/1 -> Add1/2, Product3/2  "b"
  Power1/1 -> Product/1
  Product/1 -> Gain/1
  Gain/1 -> Add/2
  Power/1 -> Add/1
  Add1/1 -> Product/2
  c/1 -> Product1/2, Product2/1  "c"
  Product1/1 -> Gain1/1
  lambda/1 -> Product1/1, Power1/1, Power/1  "lambda"
  Gain1/1 -> Add/3
  Add2/1 -> Add/4
  d/1 -> Gain2/1
  Gain2/1 -> Add2/3
  sigma/1 -> Product2/2
  Product2/1 -> Add2/2
  Product3/1 -> Add2/1
  Add/1 -> p(lambda)/1

== system mainModel/attitudeDetermination_QUATERNION/quest - shuster/newton method step-one/characteristic polynomial derivative ==
  lambda : Inport
  a : Inport  Port=2
  b : Inport  Port=3
  c : Inport  Port=4
  Add : Sum  Inputs=+++
  Add1 : Sum
  Constant1 : Constant  Value=3
  Gain : Gain  Gain=-2
  Gain1 : Gain  Gain=-1
  Gain2 : Gain  Gain=4
  Power : Math  Operator=pow
  Product : Product
  p'(lambda) : Outport
  wires:
  Constant1/1 -> Power/2
  a/1 -> Add1/1  "a"
  b/1 -> Add1/2  "b"
  Product/1 -> Gain/1
  Gain/1 -> Add/2
  Power/1 -> Gain2/1
  Add1/1 -> Product/2
  c/1 -> Gain1/1  "c"
  lambda/1 -> Power/1, Product/1  "lambda"
  Gain1/1 -> Add/3
  Add/1 -> p'(lambda)/1
  Gain2/1 -> Add/1

== system mainModel/attitudeDetermination_QUATERNION/quest - shuster/newton method step-one/newton method step-one ==
  note: lambda0 can be setted as SIGMA only if two step newton is implemented
  p(lambda) : Inport
  p'(lambda) : Inport  Port=2
  Constant : Constant  Value=init.lambda0
  Divide : Product  Inputs=*/
  Sum : Sum  Inputs=+-
  lambda1 : Outport
  wires:
  Sum/1 -> lambda1/1
  p(lambda)/1 -> Divide/1
  p'(lambda)/1 -> Divide/2
  Divide/1 -> Sum/2
  Constant/1 -> Sum/1

== system mainModel/attitudeDetermination_QUATERNION/quest - shuster/shuster parameters/Sigma ==
  S : Inport
  Add : Sum  Inputs=+++
  Gain : Gain  Gain=1/2
  Reshape : Reshape
  Selector : Selector  NumberOfDimensions=2  InputPortWidth=3  IndexOptions=Index vector (dialog),Index vector (dialog)  Indices=1,1  OutputSizes=1,1
  Selector1 : Selector  NumberOfDimensions=2  InputPortWidth=3  IndexOptions=Index vector (dialog),Index vector (dialog)  Indices=2,2  OutputSizes=1,1
  Selector2 : Selector  NumberOfDimensions=2  InputPortWidth=3  IndexOptions=Index vector (dialog),Index vector (dialog)  Indices=3,3  OutputSizes=1,1
  To Workspace5 : ToWorkspace  VariableName=sigma  SampleTime=-1
  sigma : Outport
  wires:
  Selector2/1 -> Add/3
  Selector/1 -> Add/1
  Selector1/1 -> Add/2
  S/1 -> Selector/1, Selector1/1, Selector2/1
  Add/1 -> Gain/1  "tr(S)"
  Gain/1 -> Reshape/1, sigma/1
  Reshape/1 -> To Workspace5/1

== system mainModel/attitudeDetermination_QUATERNION/quest - shuster/shuster parameters/compute Delta ==
  S : Inport
  Subsystem Reference : Subsystem  ReferencedSubsystem=matrixDeterminant
  Delta : Outport
  wires:
  Subsystem Reference/1 -> Delta/1  "det(S)"
  S/1 -> Subsystem Reference/1

== system mainModel/attitudeDetermination_QUATERNION/quest - shuster/shuster parameters/compute a ==
  sigma : Inport
  k : Inport  Port=2
  Minus : Sum  Inputs=+-
  Reshape1 : Reshape
  Square : Math  Operator=square
  To Workspace1 : ToWorkspace  VariableName=a  SampleTime=-1
  a : Outport
  wires:
  Square/1 -> Minus/1
  sigma/1 -> Square/1
  k/1 -> Minus/2
  Minus/1 -> Reshape1/1, a/1
  Reshape1/1 -> To Workspace1/1

== system mainModel/attitudeDetermination_QUATERNION/quest - shuster/shuster parameters/compute b ==
  sigma : Inport
  z : Inport  Port=2
  Add : Sum
  Reshape2 : Reshape
  Square : Math  Operator=square
  To Workspace2 : ToWorkspace  VariableName=b  SampleTime=-1
  Transpose : Math  Operator=transpose
  z^t * z : Product  Multiplication=Matrix(*)
  b : Outport
  wires:
  sigma/1 -> Square/1
  z/1 -> z^t * z/2, Transpose/1
  Transpose/1 -> z^t * z/1
  Add/1 -> Reshape2/1, b/1
  z^t * z/1 -> Add/2
  Square/1 -> Add/1
  Reshape2/1 -> To Workspace2/1

== system mainModel/attitudeDetermination_QUATERNION/quest - shuster/shuster parameters/compute c ==
  Delta : Inport
  z : Inport  Port=2
  S : Inport  Port=3
  Add : Sum
  Reshape3 : Reshape
  To Workspace3 : ToWorkspace  VariableName=c  SampleTime=-1
  Transpose : Math  Operator=transpose
  z^t *S * z : Product  Inputs=3  Multiplication=Matrix(*)
  c : Outport
  wires:
  Delta/1 -> Add/1
  S/1 -> z^t *S * z/2
  z/1 -> z^t *S * z/3, Transpose/1
  Transpose/1 -> z^t *S * z/1
  z^t *S * z/1 -> Add/2
  Add/1 -> Reshape3/1, c/1
  Reshape3/1 -> To Workspace3/1

== system mainModel/attitudeDetermination_QUATERNION/quest - shuster/shuster parameters/compute d ==
  S : Inport
  z : Inport  Port=2
  Reshape4 : Reshape
  S * S : Product  Multiplication=Matrix(*)
  To Workspace4 : ToWorkspace  VariableName=d  SampleTime=-1
  Transpose : Math  Operator=transpose
  z^t * S^2 * z : Product  Inputs=3  Multiplication=Matrix(*)
  d : Outport
  wires:
  Transpose/1 -> z^t * S^2 * z/1
  z/1 -> z^t * S^2 * z/3, Transpose/1
  S/1 -> S * S/2, S * S/1
  S * S/1 -> z^t * S^2 * z/2
  z^t * S^2 * z/1 -> Reshape4/1, d/1
  Reshape4/1 -> To Workspace4/1

== system mainModel/attitudeDetermination_QUATERNION/quest - shuster/shuster parameters/compute k ==
  S : Inport
  Add : Sum  Inputs=+++
  Add1 : Sum  Inputs=+++
  Gain : Gain  Gain=1/2
  Minus : Sum  Inputs=+-
  S * S : Product  Multiplication=Matrix(*)
  Selector : Selector  NumberOfDimensions=2  InputPortWidth=3  IndexOptions=Index vector (dialog),Index vector (dialog)  Indices=1,1  OutputSizes=1,1
  Selector1 : Selector  NumberOfDimensions=2  InputPortWidth=3  IndexOptions=Index vector (dialog),Index vector (dialog)  Indices=2,2  OutputSizes=1,1
  Selector2 : Selector  NumberOfDimensions=2  InputPortWidth=3  IndexOptions=Index vector (dialog),Index vector (dialog)  Indices=3,3  OutputSizes=1,1
  Selector3 : Selector  NumberOfDimensions=2  InputPortWidth=3  IndexOptions=Index vector (dialog),Index vector (dialog)  Indices=1,1  OutputSizes=1,1
  Selector4 : Selector  NumberOfDimensions=2  InputPortWidth=3  IndexOptions=Index vector (dialog),Index vector (dialog)  Indices=2,2  OutputSizes=1,1
  Selector5 : Selector  NumberOfDimensions=2  InputPortWidth=3  IndexOptions=Index vector (dialog),Index vector (dialog)  Indices=3,3  OutputSizes=1,1
  Square : Math  Operator=square
  k : Outport
  wires:
  S/1 -> S * S/2, S * S/1, Selector/1, Selector1/1, Selector2/1
  Selector1/1 -> Add/2
  Selector/1 -> Add/1
  Selector2/1 -> Add/3
  Add/1 -> Square/1
  Square/1 -> Minus/1  "tr(S)^2"
  Selector5/1 -> Add1/3
  Selector3/1 -> Add1/1
  Add1/1 -> Minus/2  "tr(S^2)"
  S * S/1 -> Selector3/1, Selector5/1, Selector4/1
  Selector4/1 -> Add1/2
  Minus/1 -> Gain/1
  Gain/1 -> k/1

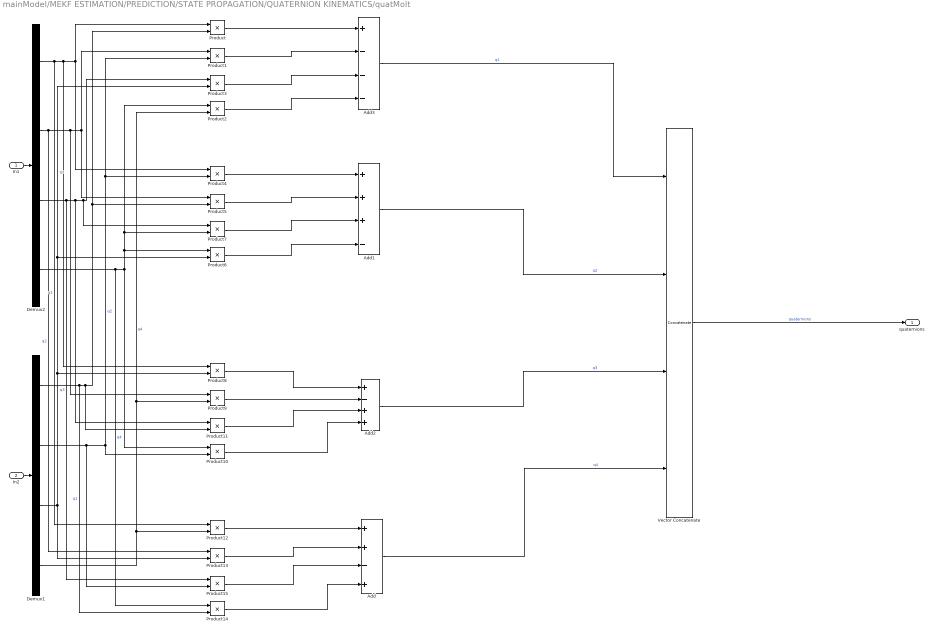
== system mainModel/MEKF ESTIMATION/PREDICTION/STATE PROPAGATION/QUATERNION KINEMATICS/quatMolt ==
  In1 : Inport
  In2 : Inport  Port=2
  Add : Sum  Inputs=++-+
  Add1 : Sum  Inputs=+++-
  Add2 : Sum  Inputs=+-++
  Add3 : Sum  Inputs=+---
  Demux1 : Demux
  Demux2 : Demux
  Product{,1..15} (16 alike) : Product
  Vector Concatenate : Concatenate  NumInputs=4
  quaternions : Outport
  wires:
  Demux1/3 -> Product13/2, Product8/2, Product6/2, Product3/2  "q3"
  Demux2/1 -> Product12/1, Product8/1, Product4/1, Product/1  "q1"
  Product/1 -> Add3/1
  Add/1 -> Vector Concatenate/4  "q4"
  Product8/1 -> Add2/1
  Demux1/2 -> Product15/2, Product10/2, Product4/2, Product1/2  "q2"
  Add1/1 -> Vector Concatenate/2  "q2"
  Demux1/1 -> Product14/2, Product11/2, Product5/2, Product/2  "q1"
  Vector Concatenate/1 -> quaternions/1  "quaternions"
  Demux2/3 -> Product15/1, Product11/1, Product7/1, Product3/1  "q3"
  Product12/1 -> Add/1
  Add2/1 -> Vector Concatenate/3  "q3"
  Product2/1 -> Add3/4
  Product1/1 -> Add3/2
  Product9/1 -> Add2/2
  Demux2/4 -> Product14/1, Product10/1, Product6/1, Product7/2, Product2/1  "q4"
  Product14/1 -> Add/4
  Demux1/4 -> Product9/2, Product2/2, Product12/2  "q4"
  Product7/1 -> Add1/3
  Product3/1 -> Add3/3
  Add3/1 -> Vector Concatenate/1  "q1"
  Product4/1 -> Add1/1
  Product6/1 -> Add1/4
  Product11/1 -> Add2/3
  In2/1 -> Demux1/1
  Demux2/2 -> Product13/1, Product9/1, Product5/1, Product1/1  "q2"
  Product13/1 -> Add/2
  Product10/1 -> Add2/4
  Product5/1 -> Add1/2
  Product15/1 -> Add/3
  In1/1 -> Demux2/1

== system mainModel/atmDrag/DRAG torque /dragForce/multipleDotProd/dotSmooth ==
  dot : Inport
  Add : Sum
  Add1 : Sum
  Constant : Constant  Value=1e-1
  Gain : Gain  Gain=1/2.2
  Sqrt : Sqrt
  Square : Math  Operator=square
  dotSmooth : Outport
  wires:
  dot/1 -> Square/1, Add/1
  Square/1 -> Add1/1
  Add1/1 -> Sqrt/1
  Constant/1 -> Add1/2
  Sqrt/1 -> Add/2
  Add/1 -> Gain/1
  Gain/1 -> dotSmooth/1

== matlab function mainModel/attitudeDetermination_QUATERNION/compute Kmatrix/MATLAB Function ==
  data: K input size=[4,4]; q_est output; lambda_max output
function [q_est, lambda_max] = quest_from_K(K)
% K: 4x4 matrix
% q_est: estimated optimal quaternion (4x1)
% lambda_max: max eigenvalue

% forcing simmetry
K = (K + K.')/2;

% computing eigenvectors and eigenvalues
[V, D] = eig(K);

% taking only real part
lambda = real(diag(D));
V      = real(V);

% finding eigenvector associated to max eigenvalue
[lambda_max, idx] = max(lambda);
q = V(:, idx);

% fixing quaternion sign
if q(1) < 0
    q = -q;
end

% normalizing the output
q_est = q / norm(q);

end

== matlab function mainModel/attitudeDetermination_QUATERNION/matlaFunction for Davenport's q-method/MATLAB Function ==
  data: K input size=[4,4]; q_est output; lambda_max output
function [q_est, lambda_max] = quest_from_K(K)
% K: 4x4 matrix
% q_est: estimated optimal quaternion (4x1)
% lambda_max: max eigenvalue

% forcing simmetry
K = (K + K.')/2;

% computing eigenvectors and eigenvalues
[V, D] = eig(K);

% taking only real part
lambda = real(diag(D));
V      = real(V);

% finding eigenvector associated to max eigenvalue
[lambda_max, idx] = max(lambda);
q = V(:, idx);

% fixing quaternion sign
if q(1) < 0
    q = -q;
end

% normalizing the output
q_est = q / norm(q);

end
